simulink model "OilT_VD"  (R2016b)
settings: configuration reference "CodeGenConfigSet" (kept outside this file)
values from neighbouring files (symbols this model uses):
  Oil_facSerPT1T_C = Calibration.Parameter    [init_OilT_VD.m]    (also in init_OilT_VD_SIL.m = Simulink.Parameter)
  Oil_RmpSlpTNeg_C = Calibration.Parameter    [init_OilT_VD.m]    (also in init_OilT_VD_SIL.m = Simulink.Parameter)
  Oil_RmpSlpTPos_C = Calibration.Parameter    [init_OilT_VD.m]    (also in init_OilT_VD_SIL.m = Simulink.Parameter)
  Oil_tDiffMaxHiT_C = Calibration.Parameter    [init_OilT_VD.m]    (also in init_OilT_VD_SIL.m = Simulink.Parameter)
  Oil_tiPlausTDefDeb_C = Calibration.Parameter    [init_OilT_VD.m]    (also in init_OilT_VD_SIL.m = Simulink.Parameter)
  Oil_tiPlausTOKDeb_C = Calibration.Parameter    [init_OilT_VD.m]    (also in init_OilT_VD_SIL.m = Simulink.Parameter)
  Oil_tTransStgTDfl_C = Calibration.Parameter    [init_OilT_VD.m]    (also in init_OilT_VD_SIL.m = Simulink.Parameter)
  SigTst_swtOilTSwmp_C = Calibration.Parameter    [init_OilT_VD.m]    (also in init_OilT_VD_SIL.m = Simulink.Parameter)
  SigTst_tOilTSwmp_C = Calibration.Parameter    [init_OilT_VD.m]    (also in init_OilT_VD_SIL.m = Simulink.Parameter)
undefined symbols (not defined in the file or in its folder): CEngDst_switch_conv, OilT_VD_DT, Switch_conv
libraries: CXLib x7
settings Model: Creator=Wollf  LastModifiedBy=lenovo
settings ConfigSetRef: SourceLocation=Base Workspace

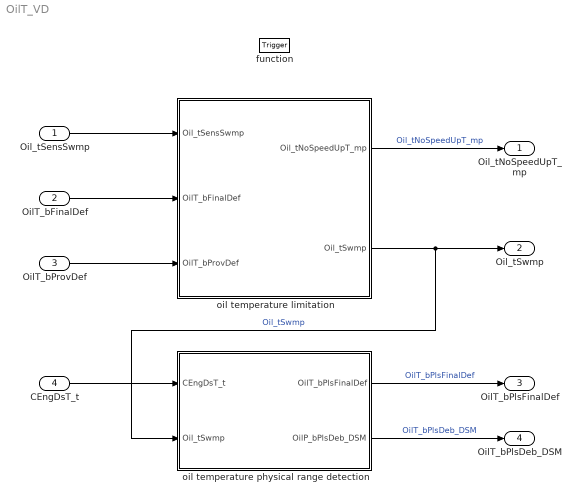
== system OilT_VD ==
  Oil_tSensSwmp : Inport  Tag=deg  Description=Sensed value of oil temperature  OutMin=-50  OutMax=200  OutDataTypeStr=Temp_deg
  OilT_bFinalDef : Inport  Description=Status Sensor of the oil temperature finally defect  Port=2  OutMin=0  OutMax=1  OutDataTypeStr=boolean
  OilT_bProvDef : Inport  Description=Status sensor of the oil temperature temporary defect  Port=3  OutMin=0  OutMax=1  OutDataTypeStr=boolean
  CEngDsT_t : Inport  Tag=deg  Description=engine coolant temperature after filter  Port=4  OutMin=-200  OutMax=200  OutDataTypeStr=Temp_deg
  function : TriggerPort  TriggerType=function-call  VariantControl=Variant
  oil temperature limitation : Subsystem
  oil temperature physical range detection : Subsystem
  Oil_tNoSpeedUpT_mp : Outport  Tag=deg  Description=Output of the trasition function without speedup  OutMin=-50  OutMax=200  OutDataTypeStr=Temp_deg
  Oil_tSwmp : Outport  Tag=deg  Description=Oil temperature in oil sump  Port=2  OutMin=-50  OutMax=200  OutDataTypeStr=Temp_deg
  OilT_bPlsFinalDef : Outport  Description=Status sensor of the oil temperature physical signal range check finally defect  Port=3  OutMin=0  OutMax=1  OutDataTypeStr=boolean
  OilT_bPlsDeb_DSM : Outport  Description=status of OilT_bPlsDeb  Port=4  OutMin=0  OutMax=1  OutDataTypeStr=boolean
  wires:
  oil temperature limitation/2(Oil_tSwmp) -> Oil_tSwmp/1, oil temperature physical range detection/2(Oil_tSwmp)  "Oil_tSwmp"
  Oil_tSensSwmp/1 -> oil temperature limitation/1(Oil_tSensSwmp)
  OilT_bFinalDef/1 -> oil temperature limitation/2(OilT_bFinalDef)
  OilT_bProvDef/1 -> oil temperature limitation/3(OilT_bProvDef)
  oil temperature limitation/1(Oil_tNoSpeedUpT_mp) -> Oil_tNoSpeedUpT_mp/1  "Oil_tNoSpeedUpT_mp"
  CEngDsT_t/1 -> oil temperature physical range detection/1(CEngDsT_t)
  oil temperature physical range detection/1(OilT_bPlsFinalDef) -> OilT_bPlsFinalDef/1  "OilT_bPlsFinalDef"
  oil temperature physical range detection/2(OilP_bPlsDeb_DSM) -> OilT_bPlsDeb_DSM/1  "OilT_bPlsDeb_DSM"

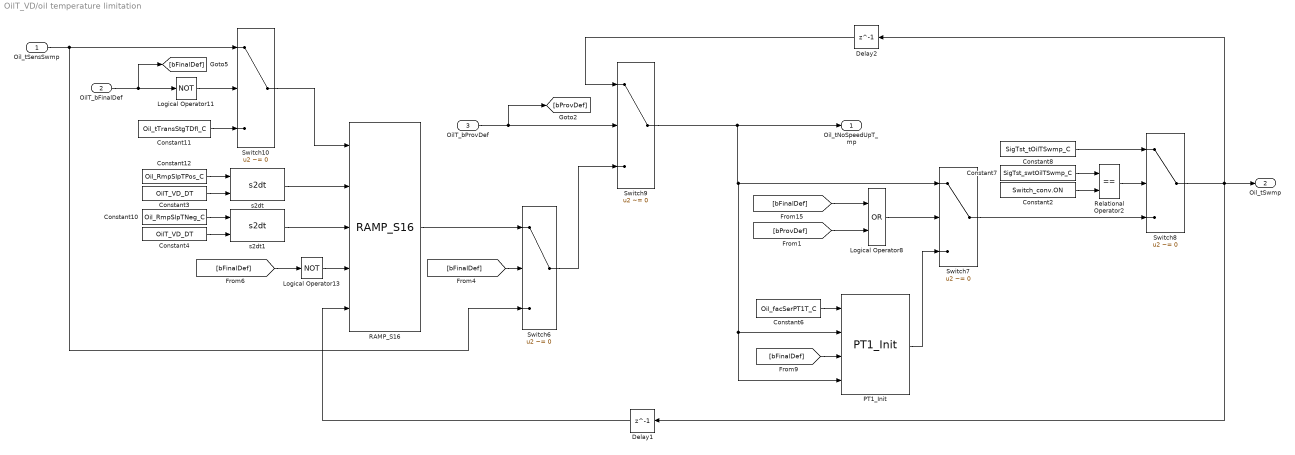
== system OilT_VD/oil temperature limitation ==
  Oil_tSensSwmp : Inport
  OilT_bFinalDef : Inport  Port=2
  OilT_bProvDef : Inport  Port=3
  Constant10 : Constant  Value=Oil_RmpSlpTNeg_C  SampleTime=-1
  Constant11 : Constant  Value=Oil_tTransStgTDfl_C  SampleTime=-1
  Constant12 : Constant  Value=Oil_RmpSlpTPos_C  SampleTime=-1
  Constant2 : Constant  Value=Switch_conv.ON  OutDataTypeStr=Inherit: Inherit via back propagation
  Constant3 : Constant  Value=OilT_VD_DT  OutDataTypeStr=int16  SampleTime=-1
  Constant4 : Constant  Value=OilT_VD_DT  OutDataTypeStr=int16  SampleTime=-1
  Constant6 : Constant  Value=Oil_facSerPT1T_C  SampleTime=-1
  Constant7 : Constant  Value=SigTst_swtOilTSwmp_C  SampleTime=-1
  Constant8 : Constant  Value=SigTst_tOilTSwmp_C  SampleTime=-1
  Delay1 : Delay  DialogController=Simulink.DDGSource  DelayLength=1  InitialCondition=0
  Delay2 : Delay  DialogController=Simulink.DDGSource  DelayLength=1  InitialCondition=0
  Logical Operator11 : Logic  Operator=NOT  AllPortsSameDT=off  OutDataTypeStr=boolean
  Logical Operator13 : Logic  Operator=NOT  AllPortsSameDT=off  OutDataTypeStr=boolean
  Logical Operator8 : Logic  Operator=OR  OutDataTypeStr=boolean
  PT1_Init : CXLib/PT1_Init  offset=2731.4
  RAMP_S16 : CXLib/RAMP_S16
  Relational Operator2 : RelationalOperator  Operator===  OutDataTypeStr=boolean  RndMeth=Simplest  InputSameDT=on
  Switch{6..7,9..10} (4 alike) : Switch  Criteria=u2 ~= 0  InputSameDT=on
  Switch8 : Switch  Criteria=u2 ~= 0  Threshold=CEngDst_switch_conv.OFF  InputSameDT=on
  s2dt : CXLib/s2dt
  s2dt1 : CXLib/s2dt
  Oil_tNoSpeedUpT_mp : Outport
  Oil_tSwmp : Outport  Port=2
  wires:
  Switch8/1 -> Oil_tSwmp/1, Delay1/1, Delay2/1
  Relational Operator2/1 -> Switch8/2
  Constant6/1 -> PT1_Init/1
  s2dt1/1 -> RAMP_S16/3
  PT1_Init/1 -> Switch7/3
  RAMP_S16/1 -> Switch6/1
  [bFinalDef] -> Logical Operator13/1
  [bFinalDef] -> Logical Operator8/1
  [bProvDef] -> Logical Operator8/2
  Logical Operator13/1 -> RAMP_S16/4
  [bFinalDef] -> Switch6/2
  [bFinalDef] -> PT1_Init/3
  Delay1/1 -> RAMP_S16/5
  Constant11/1 -> Switch10/3
  Switch7/1 -> Switch8/3
  Logical Operator8/1 -> Switch7/2
  Switch9/1 -> Oil_tNoSpeedUpT_mp/1, PT1_Init/4, PT1_Init/2, Switch7/1
  Switch6/1 -> Switch9/3
  Delay2/1 -> Switch9/1
  Oil_tSensSwmp/1 -> Switch6/3, Switch10/1
  OilT_bProvDef/1 -> [bProvDef], Switch9/2
  OilT_bFinalDef/1 -> [bFinalDef], Logical Operator11/1
  Constant10/1 -> s2dt1/1
  Constant2/1 -> Relational Operator2/2
  s2dt/1 -> RAMP_S16/2
  Constant4/1 -> s2dt1/2
  Switch10/1 -> RAMP_S16/1
  Constant12/1 -> s2dt/1
  Constant7/1 -> Relational Operator2/1
  Constant3/1 -> s2dt/2
  Logical Operator11/1 -> Switch10/2
  Constant8/1 -> Switch8/1

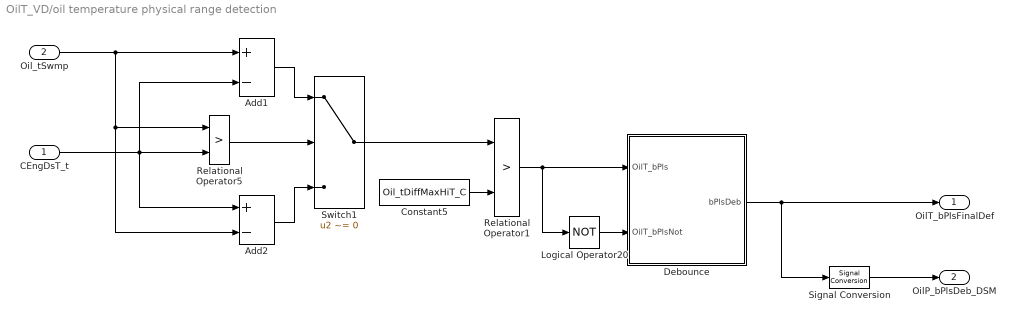
== system OilT_VD/oil temperature physical range detection ==
  CEngDsT_t : Inport
  Oil_tSwmp : Inport  Port=2
  Add1 : Sum  Inputs=+-  OutDataTypeStr=Inherit: Inherit via back propagation  InputSameDT=on
  Add2 : Sum  Inputs=+-  OutDataTypeStr=Inherit: Inherit via back propagation  InputSameDT=on
  Constant5 : Constant  Value=Oil_tDiffMaxHiT_C  SampleTime=-1
  Debounce : Subsystem
  Logical Operator20 : Logic  Operator=NOT  AllPortsSameDT=off  OutDataTypeStr=boolean
  Relational Operator1 : RelationalOperator  Operator=>  OutDataTypeStr=boolean  RndMeth=Nearest  InputSameDT=on
  Relational Operator5 : RelationalOperator  Operator=>  OutDataTypeStr=boolean  RndMeth=Nearest  InputSameDT=on
  Signal Conversion : SignalConversion  OverrideOpt=off
  Switch1 : Switch  Criteria=u2 ~= 0  InputSameDT=on
  OilT_bPlsFinalDef : Outport
  OilP_bPlsDeb_DSM : Outport  Port=2
  wires:
  Oil_tSwmp/1 -> Relational Operator5/1, Add2/2, Add1/1
  Debounce/1(bPlsDeb) -> Signal Conversion/1, OilT_bPlsFinalDef/1
  Relational Operator1/1 -> Debounce/1(OilT_bPls), Logical Operator20/1
  Logical Operator20/1 -> Debounce/2(OilT_bPlsNot)
  CEngDsT_t/1 -> Add1/2, Add2/1, Relational Operator5/2
  Switch1/1 -> Relational Operator1/1
  Add1/1 -> Switch1/1
  Relational Operator5/1 -> Switch1/2
  Constant5/1 -> Relational Operator1/2
  Add2/1 -> Switch1/3
  Signal Conversion/1 -> OilP_bPlsDeb_DSM/1

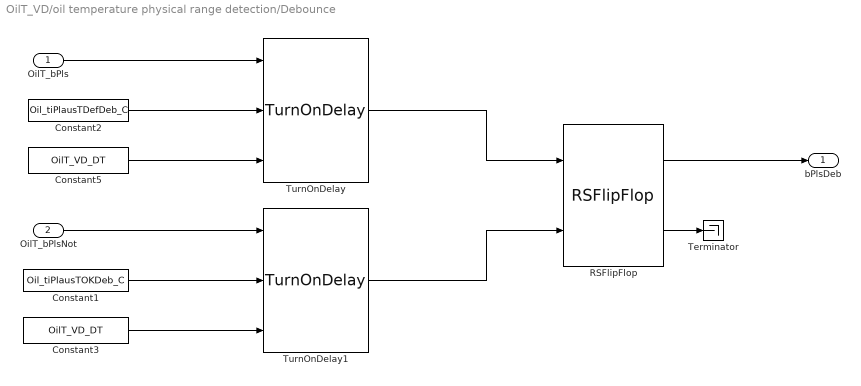
== system OilT_VD/oil temperature physical range detection/Debounce ==
  OilT_bPls : Inport
  OilT_bPlsNot : Inport  Port=2
  Constant1 : Constant  Value=Oil_tiPlausTOKDeb_C  OutDataTypeStr=Inherit: Inherit via back propagation
  Constant2 : Constant  Value=Oil_tiPlausTDefDeb_C  OutDataTypeStr=Inherit: Inherit via back propagation
  Constant3 : Constant  Value=OilT_VD_DT  OutDataTypeStr=Inherit: Inherit via back propagation  SampleTime=-1
  Constant5 : Constant  Value=OilT_VD_DT  OutDataTypeStr=Inherit: Inherit via back propagation  SampleTime=-1
  RSFlipFlop : CXLib/RSFlipFlop
  Terminator : Terminator
  TurnOnDelay : CXLib/TurnOnDelay
  TurnOnDelay1 : CXLib/TurnOnDelay
  bPlsDeb : Outport
  wires:
  OilT_bPls/1 -> TurnOnDelay/1
  RSFlipFlop/2 -> Terminator/1
  OilT_bPlsNot/1 -> TurnOnDelay1/1
  TurnOnDelay/1 -> RSFlipFlop/1
  TurnOnDelay1/1 -> RSFlipFlop/2
  RSFlipFlop/1 -> bPlsDeb/1
  Constant5/1 -> TurnOnDelay/3
  Constant3/1 -> TurnOnDelay1/3
  Constant1/1 -> TurnOnDelay1/2
  Constant2/1 -> TurnOnDelay/2
